simulink model "week1problem2"  (R2020b)
settings: Solver=VariableStepAuto  StartTime=0.0  StopTime=10.0  RelTol=1e-3
model workspace (MAT data in the model file):
  b = Simulink.Parameter
  b.Value = 3
  b.DataType = 'auto'
  b.Dimensions = [1 1]
  k = Simulink.Parameter
  k.Value = 0.01
  k.DataType = 'auto'
  k.Dimensions = [1 1]
  k1 = Simulink.Parameter
  k1.Value = 1
  k1.DataType = 'auto'
  k1.Dimensions = [1 1]
  x1_m1 = Simulink.Parameter
  x1_m1.Value = 2
  x1_m1.DataType = 'auto'
  x1_m1.Dimensions = [1 1]
  x1_m2 = 3
values from neighbouring files (symbols this model uses):
  b = 20    [Problem2nd.m]
  k1 = 50    [Problem2nd.m]
  k2 = 200    [Problem2nd.m]
  m1 = 150    [Problem2nd.m]
  m2 = 100    [Problem2nd.m]
settings Model: Creator=HP  LastModifiedBy=HP

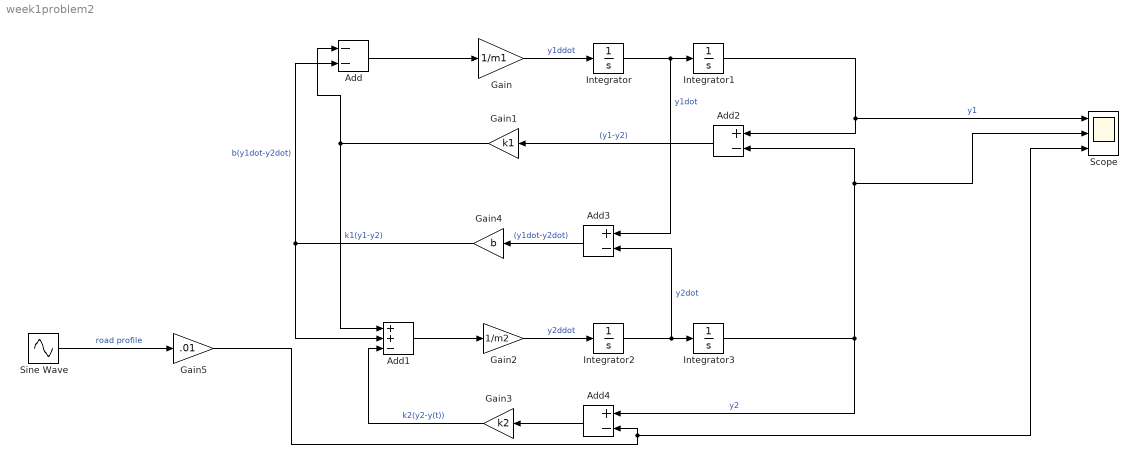
== system week1problem2 ==
  Add : Sum  Inputs=--
  Add1 : Sum  Inputs=++-
  Add2 : Sum  Inputs=+-
  Add3 : Sum  Inputs=+-
  Add4 : Sum  Inputs=+-
  Gain : Gain  Gain=1/m1
  Gain1 : Gain  Gain=k1
  Gain2 : Gain  Gain=1/m2
  Gain3 : Gain  Gain=k2
  Gain4 : Gain  Gain=b
  Gain5 : Gain  Gain=.01
  Integrator{,1..3} (4 alike) : Integrator
  Scope : Scope  NumInputPorts=3
  Sine Wave : Sin  Amplitude=2  Frequency=10  SampleTime=0
  wires:
  Gain5/1 -> Add4/2, Scope/3
  Integrator/1 -> Add3/1, Integrator1/1  "y1dot"
  Gain/1 -> Integrator/1  "y1ddot"
  Add2/1 -> Gain1/1  "(y1-y2)"
  Gain3/1 -> Add1/3  "k2(y2-y(t))"
  Integrator1/1 -> Add2/1, Scope/1  "y1"
  Sine Wave/1 -> Gain5/1  "road profile"
  Gain4/1 -> Add1/2, Add/2  "b(y1dot-y2dot)"
  Add/1 -> Gain/1
  Integrator2/1 -> Add3/2, Integrator3/1  "y2dot"
  Gain1/1 -> Add1/1, Add/1  "k1(y1-y2)"
  Integrator3/1 -> Add4/1, Scope/2, Add2/2  "y2"
  Add3/1 -> Gain4/1  "(y1dot-y2dot)"
  Add1/1 -> Gain2/1
  Add4/1 -> Gain3/1
  Gain2/1 -> Integrator2/1  "y2ddot"
